simulink model "dyn_mpc_control_sim"  (R2019b)
settings: Solver=FixedStepAuto  StartTime=0.0  StopTime=40.15  FixedStep=h  RelTol=1e-3
values from neighbouring files (symbols this model uses):
  h = 0.1    [Example_9_Tracking_Delta_Input_Formulation.m]    (also in dyn_dist_mpc_control.m = 0.01; dyn_mpc_control.m = 0.01; dyn_pid_control.m = 0.01; init.m = 0.05)
libraries: mpclib x1
settings Model: Creator=faaizz  LastModifiedBy=faaizz
settings SFSimCC: CustomCodeUndefinedFunction=UseInterfaceOnly

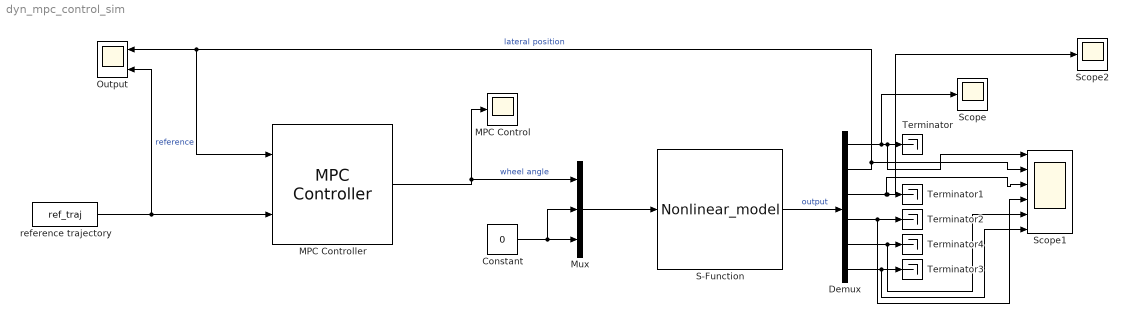
== system dyn_mpc_control_sim ==
  Constant : Constant  Value=0
  Demux : Demux  Outputs=6
  MPC Control : Scope
  MPC Controller : mpclib/MPC Controller  SCDEnableBlockLinearizationSpecification=on  mpcobj=mpcobj  is_multiple=0  enable_value=0  return_u0=off  updateMPCinCallerWorkspace=on  md_inport=off  mv_inport=off  uref_inport=off  return_cost=off  return_mvseq=off  return_qpstatus=off  return_xseq=off  return_state=off  return_ovseq=off  state_inport=off  umin_inport=off  umax_inport=off  ymin_inport=off  ymax_inport=off  cc_inport=off  ywt_inport=off  uwt_inport=off  duwt_inport=off  rhoeps_inport=off  pm_inport=off  MaximumP=10  HorizonChoice=FixedHorizon  n_ts=0.05  n_p=250  n_mv=1  n_md=0  n_ud=0  n_mo=1  n_uo=0  BlockDataType=double  SampleTimeInherited=on  switch_inport=off
  Mux : Mux  Inputs=3
  Output : Scope  NumInputPorts=2
  S-Function : S-Function  FunctionName=Nonlinear_model  SFunctionDeploymentMode=off  EnableBusSupport=off
  Scope : Scope
  Scope1 : Scope  NumInputPorts=6
  Scope2 : Scope
  Terminator{,1..4} (5 alike) : Terminator
  reference trajectory : FromWorkspace  VariableName=ref_traj  SampleTime=h  OutputAfterFinalValue=Setting to zero
  wires:
  reference trajectory/1 -> Output/2, MPC Controller/2  "reference"
  MPC Controller/1 -> MPC Control/1, Mux/1  "wheel angle"
  S-Function/1 -> Demux/1  "output"
  Mux/1 -> S-Function/1
  Constant/1 -> Mux/3, Mux/2
  Demux/2 -> Scope1/2, MPC Controller/1, Output/1  "lateral position"
  Demux/4 -> Scope1/4, Terminator2/1
  Demux/3 -> Scope2/1, Terminator1/1, Scope1/3
  Demux/1 -> Scope/1, Scope1/1, Terminator/1
  Demux/6 -> Scope1/6, Terminator3/1
  Demux/5 -> Scope1/5, Terminator4/1
